simulink model "TextsaveForSimulink"  (R2019b)
settings: Solver=VariableStepAuto  StartTime=0.0  StopTime=10.0  RelTol=1e-3
settings Model: Creator=rein  LastModifiedBy=rein

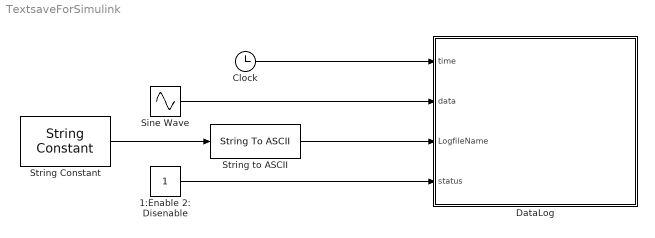
== system TextsaveForSimulink ==
  1:Enable 2: Disenable : Constant
  Clock : Clock
  DataLog : MATLAB Function  StopFcn=|  TreatAsAtomicUnit=on
      | coder.extrinsic("serial","fclose")
      | x = serial('COM3');
      | fclose(x);
  Sine Wave : Sin  SampleTime=0
  String Constant : StringConstant  String="\"Test\""
  String to ASCII : StringToASCII  OutputVectorSize=4
  wires:
  Clock/1 -> DataLog/1(time)
  Sine Wave/1 -> DataLog/2(data)
  String to ASCII/1 -> DataLog/3(LogfileName)
  1:Enable 2: Disenable/1 -> DataLog/4(status)
  String Constant/1 -> String to ASCII/1

== matlab function TextsaveForSimulink/DataLog ==
  data: time input; data input; LogfileName input; status input
function DataLog(time,data,LogfileName,status)
coder.extrinsic("sprintf");
str=sprintf("Time,%f,data,%f\r\n",time,data(1));
if status==true
    filename=char(LogfileName);
    fileID= fopen(['./' filename '.txt'],'a');
    fprintf(fileID,str);
    fclose(fileID);
end
%u=1
